simulink model "voltage_torque_mapping"  (R2023a)
settings: Solver=VariableStepAuto  StartTime=0.0  StopTime=10.0  RelTol=1e-3
values from neighbouring files (symbols this model uses):
  Ia_init = 0    [ELEN90064_Project_Parameters.m]
undefined symbols (not defined in the file or in its folder): val
settings Model: Creator=yunzh  LastModifiedBy=yunzh

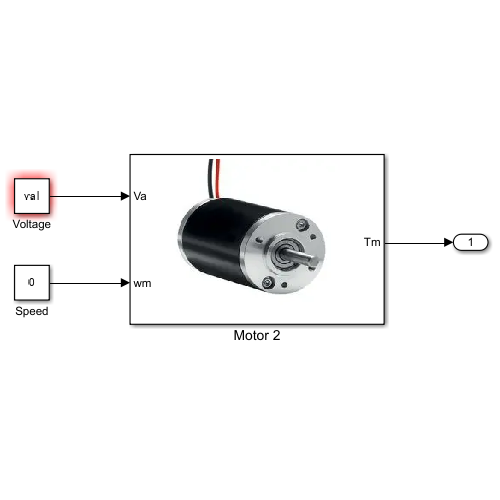
[thumbnail: Simulink's stored preview of the top-level diagram]
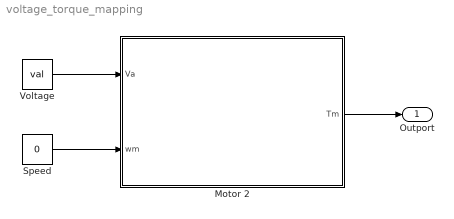
== system voltage_torque_mapping ==
  Motor 2 : Subsystem
      mask Display: image('$imagefile'); % Use "Edit Image" on toolstrip to change.
  Speed : Constant  Value=0
  Voltage : Constant  Value=val
  Outport : Outport
  wires:
  Speed/1 -> Motor 2/2(wm)
  Voltage/1 -> Motor 2/1(Va)
  Motor 2/1(Tm) -> Outport/1

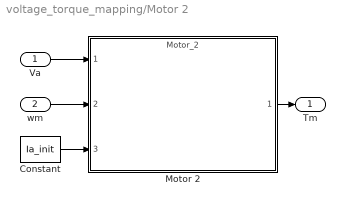
== system voltage_torque_mapping/Motor 2 ==
  Va : Inport
  wm : Inport  Port=2
  Constant : Constant  Value=Ia_init
  Motor 2 : ModelReference  ModelNameDialog=Motor_2  ModelReferenceVersion=1.19  CopyOfModelProtected=on
  Tm : Outport
  wires:
  Constant/1 -> Motor 2/3
  wm/1 -> Motor 2/2
  Va/1 -> Motor 2/1
  Motor 2/1 -> Tm/1
